simulink model "balance_robot"  (R2024a)
settings: Solver=VariableStepAuto  StartTime=0.0  StopTime=5.2  RelTol=1e-3
values from neighbouring files (symbols this model uses):
  K_cons = zeros(40,6)    [k_calc_chuan.m]    (also in k_calc_chuan_real.m; k_calc_chuanlian_simulink.m)
  X = [x1, x2, x1sq, x2sq, x1x2]    [k_calc_chuan.m]    (also in k_calc_chuan_real.m; k_calc_chuanlian_simulink.m)
undefined symbols (not defined in the file or in its folder): Y, Z
libraries: sm_lib x114, nesl_utility x19, slpidlib x3, simulink x1
(part 3 of 3)

== matlab function balance_robot/RVMC/MATLAB Function ==
  data: phi1 input; L0 output; phi4 input; phi0 output
function [L0,phi0] = L0_PHI0(phi1,phi4)
   % l5=0.108;
   %  l1=0.15;
   %  l2=0.25;
   %  l3=0.25;
   %  l4=0.15;
   %  YD = l4*sin(phi4);
   %  YB = l1*sin(phi1);
   %  XD = l5 + l4*cos(phi4);
   %  XB = l1*cos(phi1); 
   %  lBD = sqrt((XD - XB)*(XD - XB) + (YD - YB)*(YD - YB));
   %  A0 = 2*l2*(XD - XB);
   %  B0 = 2*l2*(YD - YB);
   %  C0 = l2*l2 + lBD*lBD - l3*l3;
   %  phi2 = 2*atan2((B0 + sqrt(A0*A0 + B0*B0 - C0*C0)),(A0 + C0));
   %  XC = l1*cos(phi1) + l2*cos(phi2);
   %  YC = l1*sin(phi1) + l2*sin(phi2);
   %  L0 = sqrt((XC - l5/2)*(XC - l5/2) + YC*YC);
   %  phi0=atan2(YC,(XC-l5/2));
   l1 = 0.075;
   l2 = 0.125;
   l3 = 0.125;
   l4 = 0.075;
   l5 = 0.15;
   XD = l4*cos(phi4);
   YD = l4*sin(phi4);
   XB = l1*cos(phi1);
   YB = l1*sin(phi1);
   lBD = sqrt((XD-XB)^2+(YD-YB)^2);
   A0 = 2*l2*(XD-XB);
   B0 = 2*l2*(YD - YB);
   C0 = l2*l2 + lBD*lBD - l3*l3;
   phi2 = 2*atan2((B0 - sqrt(A0*A0 + B0*B0 - C0*C0)),(A0 + C0));
   XC = (l5/l4)*(l1*cos(phi1) + l2*cos(phi2));
   YC = (l5/l4)*(l1*sin(phi1) + l2*sin(phi2));
   L0 = sqrt(XC*XC + YC*YC);
   phi0=atan2(YC,XC);

   
end

== matlab function balance_robot/Locomotion Controller/MATLAB Function ==
  data: ll input; K output; lr input; K_cons input
function K = I2K(ll, lr, K_cons)
    x = [1, ll, lr, ll^2, lr^2, ll*lr];

    % 初始化反馈矩阵 K（4行10列）
    K = zeros(4, 10);

    % 用 KK 拟合系数矩阵计算每个 K(i,j)
    for i = 1:4
        for j = 1:10
            idx = (i - 1) * 10 + j;      % 找到 K(i,j) 在 KK 中的行号
            coeffs = K_cons(idx, :);         % 拿到该 K(i,j) 的 6 个系数
            K(i, j) = coeffs * x';       % 多项式拟合结果
        end
    end
end

== matlab function balance_robot/RVMC/MATLAB Function1 ==
  data: F0 input; T1 output; Tp input; phi1 input; phi4 input; T2 output
function [T1,T2] = VMC_calc(F0,Tp,phi1,phi4)

   l1 = 0.075;
   l2 = 0.125;
   l3 = 0.125;
   l4 = 0.075;
   l5 = 0.15;

YD = l4*sin(phi4);
YB = l1*sin(phi1);
XD = l4*cos(phi4);
XB = l1*cos(phi1);
lBD = sqrt((XD - XB)*(XD - XB) + (YD - YB)*(YD - YB));
A0 = 2*l2*(XD - XB);
B0 = 2*l2*(YD - YB);
C0 = l2*l2 + lBD*lBD - l3*l3;
phi2 = 2*atan2((B0 - sqrt(A0*A0 + B0*B0 - C0*C0)),A0 + C0);
XC = (l5/l4)*(l1*cos(phi1) + l2*cos(phi2));
YC = (l5/l4)*(l1*sin(phi1) + l2*sin(phi2));
phi3 = atan2(YB-YD+l2*sin(phi2),XB-XD+l2*cos(phi2));
L0 = sqrt(XC*XC + YC*YC);
phi0 = atan2(YC,XC);
j11 = (l1*l5*sin(phi0-phi3)*sin(phi1-phi2))/(l4*sin(phi3-phi2));
j12 = (l1*l5*cos(phi0-phi3)*sin(phi1-phi2))/(L0*l4*sin(phi3-phi2));
j21 = (l5*sin(phi0-phi2)*sin(phi3-phi4))/sin(phi3-phi2);
j22 = (l5*cos(phi0-phi2)*sin(phi3-phi4))/(L0*sin(phi3-phi2));
J = [j11 j12; j21 j22];
F = [F0;Tp];
T = J * F;
T1 = T(1,1);
T2 = T(2,1);

end

== matlab function balance_robot/RVMC/MATLAB Function2 ==
  data: phi1 input; d_phi0 output; phi4 input; d_phi1 input; d_phi4 input
function d_phi0 = D_PHI0(phi1,phi4,d_phi1,d_phi4)
    l1 = 0.075;
   l2 = 0.125;
   l3 = 0.125;
   l4 = 0.075;
   l5 = 0.15;
    d_phi0 =(d_phi1*l5^2*(l2*cos(2*atan2(- (4*l2^2*(l1*cos(phi1) - l4*cos(phi4))^2 + 4*l2^2*(l1*sin(phi1) - l4*sin(phi4))^2 - ((l1*sin(phi1) - l4*sin(phi4))^2 + l2^2 - l3^2 + (l1*cos(phi1) - l4*cos(phi4))^2)^2)^(1/2) - 2*l2*(l1*sin(phi1) - l4*sin(phi4)), (l1*sin(phi1) - l4*sin(phi4))^2 - 2*l2*(l1*cos(phi1) - l4*cos(phi4)) + l2^2 - l3^2 + (l1*cos(phi1) - l4*cos(phi4))^2)) + l1*cos(phi1))^2*((l1*cos(phi1) - (2*l2*cos(2*atan2(- (4*l2^2*(l1*cos(phi1) - l4*cos(phi4))^2 + 4*l2^2*(l1*sin(phi1) - l4*sin(phi4))^2 - ((l1*sin(phi1) - l4*sin(phi4))^2 + l2^2 - l3^2 + (l1*cos(phi1) - l4*cos(phi4))^2)^2)^(1/2) - 2*l2*(l1*sin(phi1) - l4*sin(phi4)), (l1*sin(phi1) - l4*sin(phi4))^2 - 2*l2*(l1*cos(phi1) - l4*cos(phi4)) + l2^2 - l3^2 + (l1*cos(phi1) - l4*cos(phi4))^2))*((real((2*(2*l1*sin(phi1)*(l1*cos(phi1) - l4*cos(phi4)) - 2*l1*cos(phi1)*(l1*sin(phi1) - l4*sin(phi4)))*((l1*sin(phi1) - l4*sin(phi4))^2 + l2^2 - l3^2 + (l1*cos(phi1) - l4*cos(phi4))^2) - 8*l1*l2^2*sin(phi1)*(l1*cos(phi1) - l4*cos(phi4)) + 8*l1*l2^2*cos(phi1)*(l1*sin(phi1) - l4*sin(phi4)))/(4*l2^2*(l1*cos(phi1) - l4*cos(phi4))^2 + 4*l2^2*(l1*sin(phi1) - l4*sin(phi4))^2 - ((l1*sin(phi1) - l4*sin(phi4))^2 + l2^2 - l3^2 + (l1*cos(phi1) - l4*cos(phi4))^2)^2)^(1/2))/2 + 2*l1*l2*cos(phi1))/(imag((4*l2^2*(l1*cos(phi1) - l4*cos(phi4))^2 + 4*l2^2*(l1*sin(phi1) - l4*sin(phi4))^2 - ((l1*sin(phi1) - l4*sin(phi4))^2 + l2^2 - l3^2 + (l1*cos(phi1) - l4*cos(phi4))^2)^2)^(1/2)) + (l1*sin(phi1) - l4*sin(phi4))^2 - 2*l2*(l1*cos(phi1) - l4*cos(phi4)) + l2^2 - l3^2 + (l1*cos(phi1) - l4*cos(phi4))^2) - ((real((4*l2^2*(l1*cos(phi1) - l4*cos(phi4))^2 + 4*l2^2*(l1*sin(phi1) - l4*sin(phi4))^2 - ((l1*sin(phi1) - l4*sin(phi4))^2 + l2^2 - l3^2 + (l1*cos(phi1) - l4*cos(phi4))^2)^2)^(1/2)) + 2*l2*(l1*sin(phi1) - l4*sin(phi4)))*(imag((2*(2*l1*sin(phi1)*(l1*cos(phi1) - l4*cos(phi4)) - 2*l1*cos(phi1)*(l1*sin(phi1) - l4*sin(phi4)))*((l1*sin(phi1) - l4*sin(phi4))^2 + l2^2 - l3^2 + (l1*cos(phi1) - l4*cos(phi4))^2) - 8*l1*l2^2*sin(phi1)*(l1*cos(phi1) - l4*cos(phi4)) + 8*l1*l2^2*cos(phi1)*(l1*sin(phi1) - l4*sin(phi4)))/(4*l2^2*(l1*cos(phi1) - l4*cos(phi4))^2 + 4*l2^2*(l1*sin(phi1) - l4*sin(phi4))^2 - ((l1*sin(phi1) - l4*sin(phi4))^2 + l2^2 - l3^2 + (l1*cos(phi1) - l4*cos(phi4))^2)^2)^(1/2))/2 + 2*l1*l2*sin(phi1) - 2*l1*sin(phi1)*(l1*cos(phi1) - l4*cos(phi4)) + 2*l1*cos(phi1)*(l1*sin(phi1) - l4*sin(phi4))))/(imag((4*l2^2*(l1*cos(phi1) - l4*cos(phi4))^2 + 4*l2^2*(l1*sin(phi1) - l4*sin(phi4))^2 - ((l1*sin(phi1) - l4*sin(phi4))^2 + l2^2 - l3^2 + (l1*cos(phi1) - l4*cos(phi4))^2)^2)^(1/2)) + (l1*sin(phi1) - l4*sin(phi4))^2 - 2*l2*(l1*cos(phi1) - l4*cos(phi4)) + l2^2 - l3^2 + (l1*cos(phi1) - l4*cos(phi4))^2)^2)*(imag((4*l2^2*(l1*cos(phi1) - l4*cos(phi4))^2 + 4*l2^2*(l1*sin(phi1) - l4*sin(phi4))^2 - ((l1*sin(phi1) - l4*sin(phi4))^2 + l2^2 - l3^2 + (l1*cos(phi1) - l4*cos(phi4))^2)^2)^(1/2)) + (l1*sin(phi1) - l4*sin(phi4))^2 - 2*l2*(l1*cos(phi1) - l4*cos(phi4)) + l2^2 - l3^2 + (l1*cos(phi1) - l4*cos(phi4))^2)^2)/((imag((4*l2^2*(l1*cos(phi1) - l4*cos(phi4))^2 + 4*l2^2*(l1*sin(phi1) - l4*sin(phi4))^2 - ((l1*sin(phi1) - l4*sin(phi4))^2 + l2^2 - l3^2 + (l1*cos(phi1) - l4*cos(phi4))^2)^2)^(1/2)) + (l1*sin(phi1) - l4*sin(phi4))^2 - 2*l2*(l1*cos(phi1) - l4*cos(phi4)) + l2^2 - l3^2 + (l1*cos(phi1) - l4*cos(phi4))^2)^2 + (real((4*l2^2*(l1*cos(phi1) - l4*cos(phi4))^2 + 4*l2^2*(l1*sin(phi1) - l4*sin(phi4))^2 - ((l1*sin(phi1) - l4*sin(phi4))^2 + l2^2 - l3^2 + (l1*cos(phi1) - l4*cos(phi4))^2)^2)^(1/2)) + 2*l2*(l1*sin(phi1) - l4*sin(phi4)))^2))/(l2*cos(2*atan2(- (4*l2^2*(l1*cos(phi1) - l4*cos(phi4))^2 + 4*l2^2*(l1*sin(phi1) - l4*sin(phi4))^2 - ((l1*sin(phi1) - l4*sin(phi4))^2 + l2^2 - l3^2 + (l1*cos(phi1) - l4*cos(phi4))^2)^2)^(1/2) - 2*l2*(l1*sin(phi1) - l4*sin(phi4)), (l1*sin(phi1) - l4*sin(phi4))^2 - 2*l2*(l1*cos(phi1) - l4*cos(phi4)) + l2^2 - l3^2 + (l1*cos(phi1) - l4*cos(phi4))^2)) + l1*cos(phi1)) + ((l2*sin(2*atan2(- (4*l2^2*(l1*cos(phi1) - l4*cos(phi4))^2 + 4*l2^2*(l1*sin(phi1) - l4*sin(phi4))^2 - ((l1*sin(phi1) - l4*sin(phi4))^2 + l2^2 - l3^2 + (l1*cos(phi1) - l4*cos(phi4))^2)^2)^(1/2) - 2*l2*(l1*sin(phi1) - l4*sin(phi4)), (l1*sin(phi1) - l4*sin(phi4))^2 - 2*l2*(l1*cos(phi1) - l4*cos(phi4)) + l2^2 - l3^2 + (l1*cos(phi1) - l4*cos(phi4))^2)) + l1*sin(phi1))*(l1*sin(phi1) - (2*l2*sin(2*atan2(- (4*l2^2*(l1*cos(phi1) - l4*cos(phi4))^2 + 4*l2^2*(l1*sin(phi1) - l4*sin(phi4))^2 - ((l1*sin(phi1) - l4*sin(phi4))^2 + l2^2 - l3^2 + (l1*cos(phi1) - l4*cos(phi4))^2)^2)^(1/2) - 2*l2*(l1*sin(phi1) - l4*sin(phi4)), (l1*sin(phi1) - l4*sin(phi4))^2 - 2*l2*(l1*cos(phi1) - l4*cos(phi4)) + l2^2 - l3^2 + (l1*cos(phi1) - l4*cos(phi4))^2))*((real((2*(2*l1*sin(phi1)*(l1*cos(phi1) - l4*cos(phi4)) - 2*l1*cos(phi1)*(l1*sin(phi1) - l4*sin(phi4)))*((l1*sin(phi1) - l4*sin(phi4))^2 + l2^2 - l3^2 + (l1*cos(phi1) - l4*cos(phi4))^2) - 8*l1*l2^2*sin(phi1)*(l1*cos(phi1) - l4*cos(phi4)) + 8*l1*l2^2*cos(phi1)*(l1*sin(phi1) - l4*sin(phi4)))/(4*l2^2*(l1*cos(phi1) - l4*cos(phi4))^2 + 4*l2^2*(l1*sin(phi1) - l4*sin(phi4))^2 - ((l1*sin(phi1) - l4*sin(phi4))^2 + l2^2 - l3^2 + (l1*cos(phi1) - l4*cos(phi4))^2)^2)^(1/2))/2 + 2*l1*l2*cos(phi1))/(imag((4*l2^2*(l1*cos(phi1) - l4*cos(phi4))^2 + 4*l2^2*(l1*sin(phi1) - l4*sin(phi4))^2 - ((l1*sin(phi1) - l4*sin(phi4))^2 + l2^2 - l3^2 + (l1*cos(phi1) - l4*cos(phi4))^2)^2)^(1/2)) + (l1*sin(phi1) - l4*sin(phi4))^2 - 2*l2*(l1*cos(phi1) - l4*cos(phi4)) + l2^2 - l3^2 + (l1*cos(phi1) - l4*cos(phi4))^2) - ((real((4*l2^2*(l1*cos(phi1) - l4*cos(phi4))^2 + 4*l2^2*(l1*sin(phi1) - l4*sin(phi4))^2 - ((l1*sin(phi1) - l4*sin(phi4))^2 + l2^2 - l3^2 + (l1*cos(phi1) - l4*cos(phi4))^2)^2)^(1/2)) + 2*l2*(l1*sin(phi1) - l4*sin(phi4)))*(imag((2*(2*l1*sin(phi1)*(l1*cos(phi1) - l4*cos(phi4)) - 2*l1*cos(phi1)*(l1*sin(phi1) - l4*sin(phi4)))*((l1*sin(phi1) - l4*sin(phi4))^2 + l2^2 - l3^2 + (l1*cos(phi1) - l4*cos(phi4))^2) - 8*l1*l2^2*sin(phi1)*(l1*cos(phi1) - l4*cos(phi4)) + 8*l1*l2^2*cos(phi1)*(l1*sin(phi1) - l4*sin(phi4)))/(4*l2^2*(l1*cos(phi1) - l4*cos(phi4))^2 + 4*l2^2*(l1*sin(phi1) - l4*sin(phi4))^2 - ((l1*sin(phi1) - l4*sin(phi4))^2 + l2^2 - l3^2 + (l1*cos(phi1) - l4*cos(phi4))^2)^2)^(1/2))/2 + 2*l1*l2*sin(phi1) - 2*l1*sin(phi1)*(l1*cos(phi1) - l4*cos(phi4)) + 2*l1*cos(phi1)*(l1*sin(phi1) - l4*sin(phi4))))/(imag((4*l2^2*(l1*cos(phi1) - l4*cos(phi4))^2 + 4*l2^2*(l1*sin(phi1) - l4*sin(phi4))^2 - ((l1*sin(phi1) - l4*sin(phi4))^2 + l2^2 - l3^2 + (l1*cos(phi1) - l4*cos(phi4))^2)^2)^(1/2)) + (l1*sin(phi1) - l4*sin(phi4))^2 - 2*l2*(l1*cos(phi1) - l4*cos(phi4)) + l2^2 - l3^2 + (l1*cos(phi1) - l4*cos(phi4))^2)^2)*(imag((4*l2^2*(l1*cos(phi1) - l4*cos(phi4))^2 + 4*l2^2*(l1*sin(phi1) - l4*sin(phi4))^2 - ((l1*sin(phi1) - l4*sin(phi4))^2 + l2^2 - l3^2 + (l1*cos(phi1) - l4*cos(phi4))^2)^2)^(1/2)) + (l1*sin(phi1) - l4*sin(phi4))^2 - 2*l2*(l1*cos(phi1) - l4*cos(phi4)) + l2^2 - l3^2 + (l1*cos(phi1) - l4*cos(phi4))^2)^2)/((imag((4*l2^2*(l1*cos(phi1) - l4*cos(phi4))^2 + 4*l2^2*(l1*sin(phi1) - l4*sin(phi4))^2 - ((l1*sin(phi1) - l4*sin(phi4))^2 + l2^2 - l3^2 + (l1*cos(phi1) - l4*cos(phi4))^2)^2)^(1/2)) + (l1*sin(phi1) - l4*sin(phi4))^2 - 2*l2*(l1*cos(phi1) - l4*cos(phi4)) + l2^2 - l3^2 + (l1*cos(phi1) - l4*cos(phi4))^2)^2 + (real((4*l2^2*(l1*cos(phi1) - l4*cos(phi4))^2 + 4*l2^2*(l1*sin(phi1) - l4*sin(phi4))^2 - ((l1*sin(phi1) - l4*sin(phi4))^2 + l2^2 - l3^2 + (l1*cos(phi1) - l4*cos(phi4))^2)^2)^(1/2)) + 2*l2*(l1*sin(phi1) - l4*sin(phi4)))^2)))/(l2*cos(2*atan2(- (4*l2^2*(l1*cos(phi1) - l4*cos(phi4))^2 + 4*l2^2*(l1*sin(phi1) - l4*sin(phi4))^2 - ((l1*sin(phi1) - l4*sin(phi4))^2 + l2^2 - l3^2 + (l1*cos(phi1) - l4*cos(phi4))^2)^2)^(1/2) - 2*l2*(l1*sin(phi1) - l4*sin(phi4)), (l1*sin(phi1) - l4*sin(phi4))^2 - 2*l2*(l1*cos(phi1) - l4*cos(phi4)) + l2^2 - l3^2 + (l1*cos(phi1) - l4*cos(phi4))^2)) + l1*cos(phi1))^2))/(l4^2*((l5^2*(l2*cos(2*atan2(- (4*l2^2*(l1*cos(phi1) - l4*cos(phi4))^2 + 4*l2^2*(l1*sin(phi1) - l4*sin(phi4))^2 - ((l1*sin(phi1) - l4*sin(phi4))^2 + l2^2 - l3^2 + (l1*cos(phi1) - l4*cos(phi4))^2)^2)^(1/2) - 2*l2*(l1*sin(phi1) - l4*sin(phi4)), (l1*sin(phi1) - l4*sin(phi4))^2 - 2*l2*(l1*cos(phi1) - l4*cos(phi4)) + l2^2 - l3^2 + (l1*cos(phi1) - l4*cos(phi4))^2)) + l1*cos(phi1))^2)/l4^2 + (l5^2*(l2*sin(2*atan2(- (4*l2^2*(l1*cos(phi1) - l4*cos(phi4))^2 + 4*l2^2*(l1*sin(phi1) - l4*sin(phi4))^2 - ((l1*sin(phi1) - l4*sin(phi4))^2 + l2^2 - l3^2 + (l1*cos(phi1) - l4*cos(phi4))^2)^2)^(1/2) - 2*l2*(l1*sin(phi1) - l4*sin(phi4)), (l1*sin(phi1) - l4*sin(phi4))^2 - 2*l2*(l1*cos(phi1) - l4*cos(phi4)) + l2^2 - l3^2 + (l1*cos(phi1) - l4*cos(phi4))^2)) + l1*sin(phi1))^2)/l4^2)) + (d_phi4*l5^2*(l2*cos(2*atan2(- (4*l2^2*(l1*cos(phi1) - l4*cos(phi4))^2 + 4*l2^2*(l1*sin(phi1) - l4*sin(phi4))^2 - ((l1*sin(phi1) - l4*sin(phi4))^2 + l2^2 - l3^2 + (l1*cos(phi1) - l4*cos(phi4))^2)^2)^(1/2) - 2*l2*(l1*sin(phi1) - l4*sin(phi4)), (l1*sin(phi1) - l4*sin(phi4))^2 - 2*l2*(l1*cos(phi1) - l4*cos(phi4)) + l2^2 - l3^2 + (l1*cos(phi1) - l4*cos(phi4))^2)) + l1*cos(phi1))^2*((2*l2*cos(2*atan2(- (4*l2^2*(l1*cos(phi1) - l4*cos(phi4))^2 + 4*l2^2*(l1*sin(phi1) - l4*sin(phi4))^2 - ((l1*sin(phi1) - l4*sin(phi4))^2 + l2^2 - l3^2 + (l1*cos(phi1) - l4*cos(phi4))^2)^2)^(1/2) - 2*l2*(l1*sin(phi1) - l4*sin(phi4)), (l1*sin(phi1) - l4*sin(phi4))^2 - 2*l2*(l1*cos(phi1) - l4*cos(phi4)) + l2^2 - l3^2 + (l1*cos(phi1) - l4*cos(phi4))^2))*((real((2*(2*l4*sin(phi4)*(l1*cos(phi1) - l4*cos(phi4)) - 2*l4*cos(phi4)*(l1*sin(phi1) - l4*sin(phi4)))*((l1*sin(phi1) - l4*sin(phi4))^2 + l2^2 - l3^2 + (l1*cos(phi1) - l4*cos(phi4))^2) - 8*l2^2*l4*sin(phi4)*(l1*cos(phi1) - l4*cos(phi4)) + 8*l2^2*l4*cos(phi4)*(l1*sin(phi1) - l4*sin(phi4)))/(4*l2^2*(l1*cos(phi1) - l4*cos(phi4))^2 + 4*l2^2*(l1*sin(phi1) - l4*sin(phi4))^2 - ((l1*sin(phi1) - l4*sin(phi4))^2 + l2^2 - l3^2 + (l1*cos(phi1) - l4*cos(phi4))^2)^2)^(1/2))/2 + 2*l2*l4*cos(phi4))/(imag((4*l2^2*(l1*cos(phi1) - l4*cos(phi4))^2 + 4*l2^2*(l1*sin(phi1) - l4*sin(phi4))^2 - ((l1*sin(phi1) - l4*sin(phi4))^2 + l2^2 - l3^2 + (l1*cos(phi1) - l4*cos(phi4))^2)^2)^(1/2)) + (l1*sin(phi1) - l4*sin(phi4))^2 - 2*l2*(l1*cos(phi1) - l4*cos(phi4)) + l2^2 - l3^2 + (l1*cos(phi1) - l4*cos(phi4))^2) - ((real((4*l2^2*(l1*cos(phi1) - l4*cos(phi4))^2 + 4*l2^2*(l1*sin(phi1) - l4*sin(phi4))^2 - ((l1*sin(phi1) - l4*sin(phi4))^2 + l2^2 - l3^2 + (l1*cos(phi1) - l4*cos(phi4))^2)^2)^(1/2)) + 2*l2*(l1*sin(phi1) - l4*sin(phi4)))*(imag((2*(2*l4*sin(phi4)*(l1*cos(phi1) - l4*cos(phi4)) - 2*l4*cos(phi4)*(l1*sin(phi1) - l4*sin(phi4)))*((l1*sin(phi1) - l4*sin(phi4))^2 + l2^2 - l3^2 + (l1*cos(phi1) - l4*cos(phi4))^2) - 8*l2^2*l4*sin(phi4)*(l1*cos(phi1) - l4*cos(phi4)) + 8*l2^2*l4*cos(phi4)*(l1*sin(phi1) - l4*sin(phi4)))/(4*l2^2*(l1*cos(phi1) - l4*cos(phi4))^2 + 4*l2^2*(l1*sin(phi1) - l4*sin(phi4))^2 - ((l1*sin(phi1) - l4*sin(phi4))^2 + l2^2 - l3^2 + (l1*cos(phi1) - l4*cos(phi4))^2)^2)^(1/2))/2 + 2*l2*l4*sin(phi4) - 2*l4*sin(phi4)*(l1*cos(phi1) - l4*cos(phi4)) + 2*l4*cos(phi4)*(l1*sin(phi1) - l4*sin(phi4))))/(imag((4*l2^2*(l1*cos(phi1) - l4*cos(phi4))^2 + 4*l2^2*(l1*sin(phi1) - l4*sin(phi4))^2 - ((l1*sin(phi1) - l4*sin(phi4))^2 + l2^2 - l3^2 + (l1*cos(phi1) - l4*cos(phi4))^2)^2)^(1/2)) + (l1*sin(phi1) - l4*sin(phi4))^2 - 2*l2*(l1*cos(phi1) - l4*cos(phi4)) + l2^2 - l3^2 + (l1*cos(phi1) - l4*cos(phi4))^2)^2)*(imag((4*l2^2*(l1*cos(phi1) - l4*cos(phi4))^2 + 4*l2^2*(l1*sin(phi1) - l4*sin(phi4))^2 - ((l1*sin(phi1) - l4*sin(phi4))^2 + l2^2 - l3^2 + (l1*cos(phi1) - l4*cos(phi4))^2)^2)^(1/2)) + (l1*sin(phi1) - l4*sin(phi4))^2 - 2*l2*(l1*cos(phi1) - l4*cos(phi4)) + l2^2 - l3^2 + (l1*cos(phi1) - l4*cos(phi4))^2)^2)/((l2*cos(2*atan2(- (4*l2^2*(l1*cos(phi1) - l4*cos(phi4))^2 + 4*l2^2*(l1*sin(phi1) - l4*sin(phi4))^2 - ((l1*sin(phi1) - l4*sin(phi4))^2 + l2^2 - l3^2 + (l1*cos(phi1) - l4*cos(phi4))^2)^2)^(1/2) - 2*l2*(l1*sin(phi1) - l4*sin(phi4)), (l1*sin(phi1) - l4*sin(phi4))^2 - 2*l2*(l1*cos(phi1) - l4*cos(phi4)) + l2^2 - l3^2 + (l1*cos(phi1) - l4*cos(phi4))^2)) + l1*cos(phi1))*((imag((4*l2^2*(l1*cos(phi1) - l4*cos(phi4))^2 + 4*l2^2*(l1*sin(phi1) - l4*sin(phi4))^2 - ((l1*sin(phi1) - l4*sin(phi4))^2 + l2^2 - l3^2 + (l1*cos(phi1) - l4*cos(phi4))^2)^2)^(1/2)) + (l1*sin(phi1) - l4*sin(phi4))^2 - 2*l2*(l1*cos(phi1) - l4*cos(phi4)) + l2^2 - l3^2 + (l1*cos(phi1) - l4*cos(phi4))^2)^2 + (real((4*l2^2*(l1*cos(phi1) - l4*cos(phi4))^2 + 4*l2^2*(l1*sin(phi1) - l4*sin(phi4))^2 - ((l1*sin(phi1) - l4*sin(phi4))^2 + l2^2 - l3^2 + (l1*cos(phi1) - l4*cos(phi4))^2)^2)^(1/2)) + 2*l2*(l1*sin(phi1) - l4*sin(phi4)))^2)) + (2*l2*sin(2*atan2(- (4*l2^2*(l1*cos(phi1) - l4*cos(phi4))^2 + 4*l2^2*(l1*sin(phi1) - l4*sin(phi4))^2 - ((l1*sin(phi1) - l4*sin(phi4))^2 + l2^2 - l3^2 + (l1*cos(phi1) - l4*cos(phi4))^2)^2)^(1/2) - 2*l2*(l1*sin(phi1) - l4*sin(phi4)), (l1*sin(phi1) - l4*sin(phi4))^2 - 2*l2*(l1*cos(phi1) - l4*cos(phi4)) + l2^2 - l3^2 + (l1*cos(phi1) - l4*cos(phi4))^2))*(l2*sin(2*atan2(- (4*l2^2*(l1*cos(phi1) - l4*cos(phi4))^2 + 4*l2^2*(l1*sin(phi1) - l4*sin(phi4))^2 - ((l1*sin(phi1) - l4*sin(phi4))^2 + l2^2 - l3^2 + (l1*cos(phi1) - l4*cos(phi4))^2)^2)^(1/2) - 2*l2*(l1*sin(phi1) - l4*sin(phi4)), (l1*sin(phi1) - l4*sin(phi4))^2 - 2*l2*(l1*cos(phi1) - l4*cos(phi4)) + l2^2 - l3^2 + (l1*cos(phi1) - l4*cos(phi4))^2)) + l1*sin(phi1))*((real((2*(2*l4*sin(phi4)*(l1*cos(phi1) - l4*cos(phi4)) - 2*l4*cos(phi4)*(l1*sin(phi1) - l4*sin(phi4)))*((l1*sin(phi1) - l4*sin(phi4))^2 + l2^2 - l3^2 + (l1*cos(phi1) - l4*cos(phi4))^2) - 8*l2^2*l4*sin(phi4)*(l1*cos(phi1) - l4*cos(phi4)) + 8*l2^2*l4*cos(phi4)*(l1*sin(phi1) - l4*sin(phi4)))/(4*l2^2*(l1*cos(phi1) - l4*cos(phi4))^2 + 4*l2^2*(l1*sin(phi1) - l4*sin(phi4))^2 - ((l1*sin(phi1) - l4*sin(phi4))^2 + l2^2 - l3^2 + (l1*cos(phi1) - l4*cos(phi4))^2)^2)^(1/2))/2 + 2*l2*l4*cos(phi4))/(imag((4*l2^2*(l1*cos(phi1) - l4*cos(phi4))^2 + 4*l2^2*(l1*sin(phi1) - l4*sin(phi4))^2 - ((l1*sin(phi1) - l4*sin(phi4))^2 + l2^2 - l3^2 + (l1*cos(phi1) - l4*cos(phi4))^2)^2)^(1/2)) + (l1*sin(phi1) - l4*sin(phi4))^2 - 2*l2*(l1*cos(phi1) - l4*cos(phi4)) + l2^2 - l3^2 + (l1*cos(phi1) - l4*cos(phi4))^2) - ((real((4*l2^2*(l1*cos(phi1) - l4*cos(phi4))^2 + 4*l2^2*(l1*sin(phi1) - l4*sin(phi4))^2 - ((l1*sin(phi1) - l4*sin(phi4))^2 + l2^2 - l3^2 + (l1*cos(phi1) - l4*cos(phi4))^2)^2)^(1/2)) + 2*l2*(l1*sin(phi1) - l4*sin(phi4)))*(imag((2*(2*l4*sin(phi4)*(l1*cos(phi1) - l4*cos(phi4)) - 2*l4*cos(phi4)*(l1*sin(phi1) - l4*sin(phi4)))*((l1*sin(phi1) - l4*sin(phi4))^2 + l2^2 - l3^2 + (l1*cos(phi1) - l4*cos(phi4))^2) - 8*l2^2*l4*sin(phi4)*(l1*cos(phi1) - l4*cos(phi4)) + 8*l2^2*l4*cos(phi4)*(l1*sin(phi1) - l4*sin(phi4)))/(4*l2^2*(l1*cos(phi1) - l4*cos(phi4))^2 + 4*l2^2*(l1*sin(phi1) - l4*sin(phi4))^2 - ((l1*sin(phi1) - l4*sin(phi4))^2 + l2^2 - l3^2 + (l1*cos(phi1) - l4*cos(phi4))^2)^2)^(1/2))/2 + 2*l2*l4*sin(phi4) - 2*l4*sin(phi4)*(l1*cos(phi1) - l4*cos(phi4)) + 2*l4*cos(phi4)*(l1*sin(phi1) - l4*sin(phi4))))/(imag((4*l2^2*(l1*cos(phi1) - l4*cos(phi4))^2 + 4*l2^2*(l1*sin(phi1) - l4*sin(phi4))^2 - ((l1*sin(phi1) - l4*sin(phi4))^2 + l2^2 - l3^2 + (l1*cos(phi1) - l4*cos(phi4))^2)^2)^(1/2)) + (l1*sin(phi1) - l4*sin(phi4))^2 - 2*l2*(l1*cos(phi1) - l4*cos(phi4)) + l2^2 - l3^2 + (l1*cos(phi1) - l4*cos(phi4))^2)^2)*(imag((4*l2^2*(l1*cos(phi1) - l4*cos(phi4))^2 + 4*l2^2*(l1*sin(phi1) - l4*sin(phi4))^2 - ((l1*sin(phi1) - l4*sin(phi4))^2 + l2^2 - l3^2 + (l1*cos(phi1) - l4*cos(phi4))^2)^2)^(1/2)) + (l1*sin(phi1) - l4*sin(phi4))^2 - 2*l2*(l1*cos(phi1) - l4*cos(phi4)) + l2^2 - l3^2 + (l1*cos(phi1) - l4*cos(phi4))^2)^2)/((l2*cos(2*atan2(- (4*l2^2*(l1*cos(phi1) - l4*cos(phi4))^2 + 4*l2^2*(l1*sin(phi1) - l4*sin(phi4))^2 - ((l1*sin(phi1) - l4*sin(phi4))^2 + l2^2 - l3^2 + (l1*cos(phi1) - l4*cos(phi4))^2)^2)^(1/2) - 2*l2*(l1*sin(phi1) - l4*sin(phi4)), (l1*sin(phi1) - l4*sin(phi4))^2 - 2*l2*(l1*cos(phi1) - l4*cos(phi4)) + l2^2 - l3^2 + (l1*cos(phi1) - l4*cos(phi4))^2)) + l1*cos(phi1))^2*((imag((4*l2^2*(l1*cos(phi1) - l4*cos(phi4))^2 + 4*l2^2*(l1*sin(phi1) - l4*sin(phi4))^2 - ((l1*sin(phi1) - l4*sin(phi4))^2 + l2^2 - l3^2 + (l1*cos(phi1) - l4*cos(phi4))^2)^2)^(1/2)) + (l1*sin(phi1) - l4*sin(phi4))^2 - 2*l2*(l1*cos(phi1) - l4*cos(phi4)) + l2^2 - l3^2 + (l1*cos(phi1) - l4*cos(phi4))^2)^2 + (real((4*l2^2*(l1*cos(phi1) - l4*cos(phi4))^2 + 4*l2^2*(l1*sin(phi1) - l4*sin(phi4))^2 - ((l1*sin(phi1) - l4*sin(phi4))^2 + l2^2 - l3^2 + (l1*cos(phi1) - l4*cos(phi4))^2)^2)^(1/2)) + 2*l2*(l1*sin(phi1) - l4*sin(phi4)))^2))))/(l4^2*((l5^2*(l2*cos(2*atan2(- (4*l2^2*(l1*cos(phi1) - l4*cos(phi4))^2 + 4*l2^2*(l1*sin(phi1) - l4*sin(phi4))^2 - ((l1*sin(phi1) - l4*sin(phi4))^2 + l2^2 - l3^2 + (l1*cos(phi1) - l4*cos(phi4))^2)^2)^(1/2) - 2*l2*(l1*sin(phi1) - l4*sin(phi4)), (l1*sin(phi1) - l4*sin(phi4))^2 - 2*l2*(l1*cos(phi1) - l4*cos(phi4)) + l2^2 - l3^2 + (l1*cos(phi1) - l4*cos(phi4))^2)) + l1*cos(phi1))^2)/l4^2 + (l5^2*(l2*sin(2*atan2(- (4*l2^2*(l1*cos(phi1) - l4*cos(phi4))^2 + 4*l2^2*(l1*sin(phi1) - l4*sin(phi4))^2 - ((l1*sin(phi1) - l4*sin(phi4))^2 + l2^2 - l3^2 + (l1*cos(phi1) - l4*cos(phi4))^2)^2)^(1/2) - 2*l2*(l1*sin(phi1) - l4*sin(phi4)), (l1*sin(phi1) - l4*sin(phi4))^2 - 2*l2*(l1*cos(phi1) - l4*cos(phi4)) + l2^2 - l3^2 + (l1*cos(phi1) - l4*cos(phi4))^2)) + l1*sin(phi1))^2)/l4^2));
 
end

== matlab function balance_robot/LVMC/MATLAB Function ==
  data: phi1 input; L0 output; phi4 input; phi0 output
function [L0,phi0] = L0_PHI0(phi1,phi4)
   % l5=0.108;
   %  l1=0.15;
   %  l2=0.25;
   %  l3=0.25;
   %  l4=0.15;
   %  YD = l4*sin(phi4);
   %  YB = l1*sin(phi1);
   %  XD = l5 + l4*cos(phi4);
   %  XB = l1*cos(phi1); 
   %  lBD = sqrt((XD - XB)*(XD - XB) + (YD - YB)*(YD - YB));
   %  A0 = 2*l2*(XD - XB);
   %  B0 = 2*l2*(YD - YB);
   %  C0 = l2*l2 + lBD*lBD - l3*l3;
   %  phi2 = 2*atan2((B0 + sqrt(A0*A0 + B0*B0 - C0*C0)),(A0 + C0));
   %  XC = l1*cos(phi1) + l2*cos(phi2);
   %  YC = l1*sin(phi1) + l2*sin(phi2);
   %  L0 = sqrt((XC - l5/2)*(XC - l5/2) + YC*YC);
   %  phi0=atan2(YC,(XC-l5/2));
   l1 = 0.075;
   l2 = 0.125;
   l3 = 0.125;
   l4 = 0.075;
   l5 = 0.15;
   XD = l4*cos(phi4);
   YD = l4*sin(phi4);
   XB = l1*cos(phi1);
   YB = l1*sin(phi1);
   lBD = sqrt((XD-XB)^2+(YD-YB)^2);
   A0 = 2*l2*(XD-XB);
   B0 = 2*l2*(YD - YB);
   C0 = l2*l2 + lBD*lBD - l3*l3;
   phi2 = 2*atan2((B0 - sqrt(A0*A0 + B0*B0 - C0*C0)),(A0 + C0));
   XC = l5/l4*(l1*cos(phi1) + l2*cos(phi2));
   YC = l5/l4*(l1*sin(phi1) + l2*sin(phi2));
   L0 = sqrt(XC*XC + YC*YC);
   phi0=atan2(YC,XC);

   
end

== matlab function balance_robot/LVMC/MATLAB Function1 ==
  data: F0 input; T1 output; Tp input; phi1 input; phi4 input; T2 output
function [T1,T2] = VMC_calc(F0,Tp,phi1,phi4)

   l1 = 0.075;
   l2 = 0.125;
   l3 = 0.125;
   l4 = 0.075;
   l5 = 0.15;

YD = l4*sin(phi4);
YB = l1*sin(phi1);
XD = l4*cos(phi4);
XB = l1*cos(phi1);
lBD = sqrt((XD - XB)*(XD - XB) + (YD - YB)*(YD - YB));
A0 = 2*l2*(XD - XB);
B0 = 2*l2*(YD - YB);
C0 = l2*l2 + lBD*lBD - l3*l3;
phi2 = 2*atan2((B0 - sqrt(A0*A0 + B0*B0 - C0*C0)),A0 + C0);
XC = l5/l4*(l1*cos(phi1) + l2*cos(phi2));
YC = l5/l4*(l1*sin(phi1) + l2*sin(phi2));
phi3 = atan2(YB-YD+l2*sin(phi2),XB-XD+l2*cos(phi2));
L0 = sqrt(XC*XC + YC*YC);
phi0 = atan2(YC,XC);
j11 = (l1*l5*sin(phi0-phi3)*sin(phi1-phi2))/(l4*sin(phi3-phi2));
j12 = (l1*l5*cos(phi0-phi3)*sin(phi1-phi2))/(L0*l4*sin(phi3-phi2));
j21 = (l5*sin(phi0-phi2)*sin(phi3-phi4))/sin(phi3-phi2);
j22 = (l5*cos(phi0-phi2)*sin(phi3-phi4))/(L0*sin(phi3-phi2));
J = [j11 j12; j21 j22];
F = [F0;Tp];
T = J * F;
T1 = T(1,1);
T2 = T(2,1);

end

== matlab function balance_robot/LVMC/MATLAB Function2 ==
  data: phi1 input; d_phi0 output; phi4 input; d_phi1 input; d_phi4 input
function d_phi0 = D_PHI0(phi1,phi4,d_phi1,d_phi4)
    l1 = 0.075;
   l2 = 0.125;
   l3 = 0.125;
   l4 = 0.075;
   l5 = 0.15;
    d_phi0 =(d_phi1*l5^2*(l2*cos(2*atan2(- (4*l2^2*(l1*cos(phi1) - l4*cos(phi4))^2 + 4*l2^2*(l1*sin(phi1) - l4*sin(phi4))^2 - ((l1*sin(phi1) - l4*sin(phi4))^2 + l2^2 - l3^2 + (l1*cos(phi1) - l4*cos(phi4))^2)^2)^(1/2) - 2*l2*(l1*sin(phi1) - l4*sin(phi4)), (l1*sin(phi1) - l4*sin(phi4))^2 - 2*l2*(l1*cos(phi1) - l4*cos(phi4)) + l2^2 - l3^2 + (l1*cos(phi1) - l4*cos(phi4))^2)) + l1*cos(phi1))^2*((l1*cos(phi1) - (2*l2*cos(2*atan2(- (4*l2^2*(l1*cos(phi1) - l4*cos(phi4))^2 + 4*l2^2*(l1*sin(phi1) - l4*sin(phi4))^2 - ((l1*sin(phi1) - l4*sin(phi4))^2 + l2^2 - l3^2 + (l1*cos(phi1) - l4*cos(phi4))^2)^2)^(1/2) - 2*l2*(l1*sin(phi1) - l4*sin(phi4)), (l1*sin(phi1) - l4*sin(phi4))^2 - 2*l2*(l1*cos(phi1) - l4*cos(phi4)) + l2^2 - l3^2 + (l1*cos(phi1) - l4*cos(phi4))^2))*((real((2*(2*l1*sin(phi1)*(l1*cos(phi1) - l4*cos(phi4)) - 2*l1*cos(phi1)*(l1*sin(phi1) - l4*sin(phi4)))*((l1*sin(phi1) - l4*sin(phi4))^2 + l2^2 - l3^2 + (l1*cos(phi1) - l4*cos(phi4))^2) - 8*l1*l2^2*sin(phi1)*(l1*cos(phi1) - l4*cos(phi4)) + 8*l1*l2^2*cos(phi1)*(l1*sin(phi1) - l4*sin(phi4)))/(4*l2^2*(l1*cos(phi1) - l4*cos(phi4))^2 + 4*l2^2*(l1*sin(phi1) - l4*sin(phi4))^2 - ((l1*sin(phi1) - l4*sin(phi4))^2 + l2^2 - l3^2 + (l1*cos(phi1) - l4*cos(phi4))^2)^2)^(1/2))/2 + 2*l1*l2*cos(phi1))/(imag((4*l2^2*(l1*cos(phi1) - l4*cos(phi4))^2 + 4*l2^2*(l1*sin(phi1) - l4*sin(phi4))^2 - ((l1*sin(phi1) - l4*sin(phi4))^2 + l2^2 - l3^2 + (l1*cos(phi1) - l4*cos(phi4))^2)^2)^(1/2)) + (l1*sin(phi1) - l4*sin(phi4))^2 - 2*l2*(l1*cos(phi1) - l4*cos(phi4)) + l2^2 - l3^2 + (l1*cos(phi1) - l4*cos(phi4))^2) - ((real((4*l2^2*(l1*cos(phi1) - l4*cos(phi4))^2 + 4*l2^2*(l1*sin(phi1) - l4*sin(phi4))^2 - ((l1*sin(phi1) - l4*sin(phi4))^2 + l2^2 - l3^2 + (l1*cos(phi1) - l4*cos(phi4))^2)^2)^(1/2)) + 2*l2*(l1*sin(phi1) - l4*sin(phi4)))*(imag((2*(2*l1*sin(phi1)*(l1*cos(phi1) - l4*cos(phi4)) - 2*l1*cos(phi1)*(l1*sin(phi1) - l4*sin(phi4)))*((l1*sin(phi1) - l4*sin(phi4))^2 + l2^2 - l3^2 + (l1*cos(phi1) - l4*cos(phi4))^2) - 8*l1*l2^2*sin(phi1)*(l1*cos(phi1) - l4*cos(phi4)) + 8*l1*l2^2*cos(phi1)*(l1*sin(phi1) - l4*sin(phi4)))/(4*l2^2*(l1*cos(phi1) - l4*cos(phi4))^2 + 4*l2^2*(l1*sin(phi1) - l4*sin(phi4))^2 - ((l1*sin(phi1) - l4*sin(phi4))^2 + l2^2 - l3^2 + (l1*cos(phi1) - l4*cos(phi4))^2)^2)^(1/2))/2 + 2*l1*l2*sin(phi1) - 2*l1*sin(phi1)*(l1*cos(phi1) - l4*cos(phi4)) + 2*l1*cos(phi1)*(l1*sin(phi1) - l4*sin(phi4))))/(imag((4*l2^2*(l1*cos(phi1) - l4*cos(phi4))^2 + 4*l2^2*(l1*sin(phi1) - l4*sin(phi4))^2 - ((l1*sin(phi1) - l4*sin(phi4))^2 + l2^2 - l3^2 + (l1*cos(phi1) - l4*cos(phi4))^2)^2)^(1/2)) + (l1*sin(phi1) - l4*sin(phi4))^2 - 2*l2*(l1*cos(phi1) - l4*cos(phi4)) + l2^2 - l3^2 + (l1*cos(phi1) - l4*cos(phi4))^2)^2)*(imag((4*l2^2*(l1*cos(phi1) - l4*cos(phi4))^2 + 4*l2^2*(l1*sin(phi1) - l4*sin(phi4))^2 - ((l1*sin(phi1) - l4*sin(phi4))^2 + l2^2 - l3^2 + (l1*cos(phi1) - l4*cos(phi4))^2)^2)^(1/2)) + (l1*sin(phi1) - l4*sin(phi4))^2 - 2*l2*(l1*cos(phi1) - l4*cos(phi4)) + l2^2 - l3^2 + (l1*cos(phi1) - l4*cos(phi4))^2)^2)/((imag((4*l2^2*(l1*cos(phi1) - l4*cos(phi4))^2 + 4*l2^2*(l1*sin(phi1) - l4*sin(phi4))^2 - ((l1*sin(phi1) - l4*sin(phi4))^2 + l2^2 - l3^2 + (l1*cos(phi1) - l4*cos(phi4))^2)^2)^(1/2)) + (l1*sin(phi1) - l4*sin(phi4))^2 - 2*l2*(l1*cos(phi1) - l4*cos(phi4)) + l2^2 - l3^2 + (l1*cos(phi1) - l4*cos(phi4))^2)^2 + (real((4*l2^2*(l1*cos(phi1) - l4*cos(phi4))^2 + 4*l2^2*(l1*sin(phi1) - l4*sin(phi4))^2 - ((l1*sin(phi1) - l4*sin(phi4))^2 + l2^2 - l3^2 + (l1*cos(phi1) - l4*cos(phi4))^2)^2)^(1/2)) + 2*l2*(l1*sin(phi1) - l4*sin(phi4)))^2))/(l2*cos(2*atan2(- (4*l2^2*(l1*cos(phi1) - l4*cos(phi4))^2 + 4*l2^2*(l1*sin(phi1) - l4*sin(phi4))^2 - ((l1*sin(phi1) - l4*sin(phi4))^2 + l2^2 - l3^2 + (l1*cos(phi1) - l4*cos(phi4))^2)^2)^(1/2) - 2*l2*(l1*sin(phi1) - l4*sin(phi4)), (l1*sin(phi1) - l4*sin(phi4))^2 - 2*l2*(l1*cos(phi1) - l4*cos(phi4)) + l2^2 - l3^2 + (l1*cos(phi1) - l4*cos(phi4))^2)) + l1*cos(phi1)) + ((l2*sin(2*atan2(- (4*l2^2*(l1*cos(phi1) - l4*cos(phi4))^2 + 4*l2^2*(l1*sin(phi1) - l4*sin(phi4))^2 - ((l1*sin(phi1) - l4*sin(phi4))^2 + l2^2 - l3^2 + (l1*cos(phi1) - l4*cos(phi4))^2)^2)^(1/2) - 2*l2*(l1*sin(phi1) - l4*sin(phi4)), (l1*sin(phi1) - l4*sin(phi4))^2 - 2*l2*(l1*cos(phi1) - l4*cos(phi4)) + l2^2 - l3^2 + (l1*cos(phi1) - l4*cos(phi4))^2)) + l1*sin(phi1))*(l1*sin(phi1) - (2*l2*sin(2*atan2(- (4*l2^2*(l1*cos(phi1) - l4*cos(phi4))^2 + 4*l2^2*(l1*sin(phi1) - l4*sin(phi4))^2 - ((l1*sin(phi1) - l4*sin(phi4))^2 + l2^2 - l3^2 + (l1*cos(phi1) - l4*cos(phi4))^2)^2)^(1/2) - 2*l2*(l1*sin(phi1) - l4*sin(phi4)), (l1*sin(phi1) - l4*sin(phi4))^2 - 2*l2*(l1*cos(phi1) - l4*cos(phi4)) + l2^2 - l3^2 + (l1*cos(phi1) - l4*cos(phi4))^2))*((real((2*(2*l1*sin(phi1)*(l1*cos(phi1) - l4*cos(phi4)) - 2*l1*cos(phi1)*(l1*sin(phi1) - l4*sin(phi4)))*((l1*sin(phi1) - l4*sin(phi4))^2 + l2^2 - l3^2 + (l1*cos(phi1) - l4*cos(phi4))^2) - 8*l1*l2^2*sin(phi1)*(l1*cos(phi1) - l4*cos(phi4)) + 8*l1*l2^2*cos(phi1)*(l1*sin(phi1) - l4*sin(phi4)))/(4*l2^2*(l1*cos(phi1) - l4*cos(phi4))^2 + 4*l2^2*(l1*sin(phi1) - l4*sin(phi4))^2 - ((l1*sin(phi1) - l4*sin(phi4))^2 + l2^2 - l3^2 + (l1*cos(phi1) - l4*cos(phi4))^2)^2)^(1/2))/2 + 2*l1*l2*cos(phi1))/(imag((4*l2^2*(l1*cos(phi1) - l4*cos(phi4))^2 + 4*l2^2*(l1*sin(phi1) - l4*sin(phi4))^2 - ((l1*sin(phi1) - l4*sin(phi4))^2 + l2^2 - l3^2 + (l1*cos(phi1) - l4*cos(phi4))^2)^2)^(1/2)) + (l1*sin(phi1) - l4*sin(phi4))^2 - 2*l2*(l1*cos(phi1) - l4*cos(phi4)) + l2^2 - l3^2 + (l1*cos(phi1) - l4*cos(phi4))^2) - ((real((4*l2^2*(l1*cos(phi1) - l4*cos(phi4))^2 + 4*l2^2*(l1*sin(phi1) - l4*sin(phi4))^2 - ((l1*sin(phi1) - l4*sin(phi4))^2 + l2^2 - l3^2 + (l1*cos(phi1) - l4*cos(phi4))^2)^2)^(1/2)) + 2*l2*(l1*sin(phi1) - l4*sin(phi4)))*(imag((2*(2*l1*sin(phi1)*(l1*cos(phi1) - l4*cos(phi4)) - 2*l1*cos(phi1)*(l1*sin(phi1) - l4*sin(phi4)))*((l1*sin(phi1) - l4*sin(phi4))^2 + l2^2 - l3^2 + (l1*cos(phi1) - l4*cos(phi4))^2) - 8*l1*l2^2*sin(phi1)*(l1*cos(phi1) - l4*cos(phi4)) + 8*l1*l2^2*cos(phi1)*(l1*sin(phi1) - l4*sin(phi4)))/(4*l2^2*(l1*cos(phi1) - l4*cos(phi4))^2 + 4*l2^2*(l1*sin(phi1) - l4*sin(phi4))^2 - ((l1*sin(phi1) - l4*sin(phi4))^2 + l2^2 - l3^2 + (l1*cos(phi1) - l4*cos(phi4))^2)^2)^(1/2))/2 + 2*l1*l2*sin(phi1) - 2*l1*sin(phi1)*(l1*cos(phi1) - l4*cos(phi4)) + 2*l1*cos(phi1)*(l1*sin(phi1) - l4*sin(phi4))))/(imag((4*l2^2*(l1*cos(phi1) - l4*cos(phi4))^2 + 4*l2^2*(l1*sin(phi1) - l4*sin(phi4))^2 - ((l1*sin(phi1) - l4*sin(phi4))^2 + l2^2 - l3^2 + (l1*cos(phi1) - l4*cos(phi4))^2)^2)^(1/2)) + (l1*sin(phi1) - l4*sin(phi4))^2 - 2*l2*(l1*cos(phi1) - l4*cos(phi4)) + l2^2 - l3^2 + (l1*cos(phi1) - l4*cos(phi4))^2)^2)*(imag((4*l2^2*(l1*cos(phi1) - l4*cos(phi4))^2 + 4*l2^2*(l1*sin(phi1) - l4*sin(phi4))^2 - ((l1*sin(phi1) - l4*sin(phi4))^2 + l2^2 - l3^2 + (l1*cos(phi1) - l4*cos(phi4))^2)^2)^(1/2)) + (l1*sin(phi1) - l4*sin(phi4))^2 - 2*l2*(l1*cos(phi1) - l4*cos(phi4)) + l2^2 - l3^2 + (l1*cos(phi1) - l4*cos(phi4))^2)^2)/((imag((4*l2^2*(l1*cos(phi1) - l4*cos(phi4))^2 + 4*l2^2*(l1*sin(phi1) - l4*sin(phi4))^2 - ((l1*sin(phi1) - l4*sin(phi4))^2 + l2^2 - l3^2 + (l1*cos(phi1) - l4*cos(phi4))^2)^2)^(1/2)) + (l1*sin(phi1) - l4*sin(phi4))^2 - 2*l2*(l1*cos(phi1) - l4*cos(phi4)) + l2^2 - l3^2 + (l1*cos(phi1) - l4*cos(phi4))^2)^2 + (real((4*l2^2*(l1*cos(phi1) - l4*cos(phi4))^2 + 4*l2^2*(l1*sin(phi1) - l4*sin(phi4))^2 - ((l1*sin(phi1) - l4*sin(phi4))^2 + l2^2 - l3^2 + (l1*cos(phi1) - l4*cos(phi4))^2)^2)^(1/2)) + 2*l2*(l1*sin(phi1) - l4*sin(phi4)))^2)))/(l2*cos(2*atan2(- (4*l2^2*(l1*cos(phi1) - l4*cos(phi4))^2 + 4*l2^2*(l1*sin(phi1) - l4*sin(phi4))^2 - ((l1*sin(phi1) - l4*sin(phi4))^2 + l2^2 - l3^2 + (l1*cos(phi1) - l4*cos(phi4))^2)^2)^(1/2) - 2*l2*(l1*sin(phi1) - l4*sin(phi4)), (l1*sin(phi1) - l4*sin(phi4))^2 - 2*l2*(l1*cos(phi1) - l4*cos(phi4)) + l2^2 - l3^2 + (l1*cos(phi1) - l4*cos(phi4))^2)) + l1*cos(phi1))^2))/(l4^2*((l5^2*(l2*cos(2*atan2(- (4*l2^2*(l1*cos(phi1) - l4*cos(phi4))^2 + 4*l2^2*(l1*sin(phi1) - l4*sin(phi4))^2 - ((l1*sin(phi1) - l4*sin(phi4))^2 + l2^2 - l3^2 + (l1*cos(phi1) - l4*cos(phi4))^2)^2)^(1/2) - 2*l2*(l1*sin(phi1) - l4*sin(phi4)), (l1*sin(phi1) - l4*sin(phi4))^2 - 2*l2*(l1*cos(phi1) - l4*cos(phi4)) + l2^2 - l3^2 + (l1*cos(phi1) - l4*cos(phi4))^2)) + l1*cos(phi1))^2)/l4^2 + (l5^2*(l2*sin(2*atan2(- (4*l2^2*(l1*cos(phi1) - l4*cos(phi4))^2 + 4*l2^2*(l1*sin(phi1) - l4*sin(phi4))^2 - ((l1*sin(phi1) - l4*sin(phi4))^2 + l2^2 - l3^2 + (l1*cos(phi1) - l4*cos(phi4))^2)^2)^(1/2) - 2*l2*(l1*sin(phi1) - l4*sin(phi4)), (l1*sin(phi1) - l4*sin(phi4))^2 - 2*l2*(l1*cos(phi1) - l4*cos(phi4)) + l2^2 - l3^2 + (l1*cos(phi1) - l4*cos(phi4))^2)) + l1*sin(phi1))^2)/l4^2)) + (d_phi4*l5^2*(l2*cos(2*atan2(- (4*l2^2*(l1*cos(phi1) - l4*cos(phi4))^2 + 4*l2^2*(l1*sin(phi1) - l4*sin(phi4))^2 - ((l1*sin(phi1) - l4*sin(phi4))^2 + l2^2 - l3^2 + (l1*cos(phi1) - l4*cos(phi4))^2)^2)^(1/2) - 2*l2*(l1*sin(phi1) - l4*sin(phi4)), (l1*sin(phi1) - l4*sin(phi4))^2 - 2*l2*(l1*cos(phi1) - l4*cos(phi4)) + l2^2 - l3^2 + (l1*cos(phi1) - l4*cos(phi4))^2)) + l1*cos(phi1))^2*((2*l2*cos(2*atan2(- (4*l2^2*(l1*cos(phi1) - l4*cos(phi4))^2 + 4*l2^2*(l1*sin(phi1) - l4*sin(phi4))^2 - ((l1*sin(phi1) - l4*sin(phi4))^2 + l2^2 - l3^2 + (l1*cos(phi1) - l4*cos(phi4))^2)^2)^(1/2) - 2*l2*(l1*sin(phi1) - l4*sin(phi4)), (l1*sin(phi1) - l4*sin(phi4))^2 - 2*l2*(l1*cos(phi1) - l4*cos(phi4)) + l2^2 - l3^2 + (l1*cos(phi1) - l4*cos(phi4))^2))*((real((2*(2*l4*sin(phi4)*(l1*cos(phi1) - l4*cos(phi4)) - 2*l4*cos(phi4)*(l1*sin(phi1) - l4*sin(phi4)))*((l1*sin(phi1) - l4*sin(phi4))^2 + l2^2 - l3^2 + (l1*cos(phi1) - l4*cos(phi4))^2) - 8*l2^2*l4*sin(phi4)*(l1*cos(phi1) - l4*cos(phi4)) + 8*l2^2*l4*cos(phi4)*(l1*sin(phi1) - l4*sin(phi4)))/(4*l2^2*(l1*cos(phi1) - l4*cos(phi4))^2 + 4*l2^2*(l1*sin(phi1) - l4*sin(phi4))^2 - ((l1*sin(phi1) - l4*sin(phi4))^2 + l2^2 - l3^2 + (l1*cos(phi1) - l4*cos(phi4))^2)^2)^(1/2))/2 + 2*l2*l4*cos(phi4))/(imag((4*l2^2*(l1*cos(phi1) - l4*cos(phi4))^2 + 4*l2^2*(l1*sin(phi1) - l4*sin(phi4))^2 - ((l1*sin(phi1) - l4*sin(phi4))^2 + l2^2 - l3^2 + (l1*cos(phi1) - l4*cos(phi4))^2)^2)^(1/2)) + (l1*sin(phi1) - l4*sin(phi4))^2 - 2*l2*(l1*cos(phi1) - l4*cos(phi4)) + l2^2 - l3^2 + (l1*cos(phi1) - l4*cos(phi4))^2) - ((real((4*l2^2*(l1*cos(phi1) - l4*cos(phi4))^2 + 4*l2^2*(l1*sin(phi1) - l4*sin(phi4))^2 - ((l1*sin(phi1) - l4*sin(phi4))^2 + l2^2 - l3^2 + (l1*cos(phi1) - l4*cos(phi4))^2)^2)^(1/2)) + 2*l2*(l1*sin(phi1) - l4*sin(phi4)))*(imag((2*(2*l4*sin(phi4)*(l1*cos(phi1) - l4*cos(phi4)) - 2*l4*cos(phi4)*(l1*sin(phi1) - l4*sin(phi4)))*((l1*sin(phi1) - l4*sin(phi4))^2 + l2^2 - l3^2 + (l1*cos(phi1) - l4*cos(phi4))^2) - 8*l2^2*l4*sin(phi4)*(l1*cos(phi1) - l4*cos(phi4)) + 8*l2^2*l4*cos(phi4)*(l1*sin(phi1) - l4*sin(phi4)))/(4*l2^2*(l1*cos(phi1) - l4*cos(phi4))^2 + 4*l2^2*(l1*sin(phi1) - l4*sin(phi4))^2 - ((l1*sin(phi1) - l4*sin(phi4))^2 + l2^2 - l3^2 + (l1*cos(phi1) - l4*cos(phi4))^2)^2)^(1/2))/2 + 2*l2*l4*sin(phi4) - 2*l4*sin(phi4)*(l1*cos(phi1) - l4*cos(phi4)) + 2*l4*cos(phi4)*(l1*sin(phi1) - l4*sin(phi4))))/(imag((4*l2^2*(l1*cos(phi1) - l4*cos(phi4))^2 + 4*l2^2*(l1*sin(phi1) - l4*sin(phi4))^2 - ((l1*sin(phi1) - l4*sin(phi4))^2 + l2^2 - l3^2 + (l1*cos(phi1) - l4*cos(phi4))^2)^2)^(1/2)) + (l1*sin(phi1) - l4*sin(phi4))^2 - 2*l2*(l1*cos(phi1) - l4*cos(phi4)) + l2^2 - l3^2 + (l1*cos(phi1) - l4*cos(phi4))^2)^2)*(imag((4*l2^2*(l1*cos(phi1) - l4*cos(phi4))^2 + 4*l2^2*(l1*sin(phi1) - l4*sin(phi4))^2 - ((l1*sin(phi1) - l4*sin(phi4))^2 + l2^2 - l3^2 + (l1*cos(phi1) - l4*cos(phi4))^2)^2)^(1/2)) + (l1*sin(phi1) - l4*sin(phi4))^2 - 2*l2*(l1*cos(phi1) - l4*cos(phi4)) + l2^2 - l3^2 + (l1*cos(phi1) - l4*cos(phi4))^2)^2)/((l2*cos(2*atan2(- (4*l2^2*(l1*cos(phi1) - l4*cos(phi4))^2 + 4*l2^2*(l1*sin(phi1) - l4*sin(phi4))^2 - ((l1*sin(phi1) - l4*sin(phi4))^2 + l2^2 - l3^2 + (l1*cos(phi1) - l4*cos(phi4))^2)^2)^(1/2) - 2*l2*(l1*sin(phi1) - l4*sin(phi4)), (l1*sin(phi1) - l4*sin(phi4))^2 - 2*l2*(l1*cos(phi1) - l4*cos(phi4)) + l2^2 - l3^2 + (l1*cos(phi1) - l4*cos(phi4))^2)) + l1*cos(phi1))*((imag((4*l2^2*(l1*cos(phi1) - l4*cos(phi4))^2 + 4*l2^2*(l1*sin(phi1) - l4*sin(phi4))^2 - ((l1*sin(phi1) - l4*sin(phi4))^2 + l2^2 - l3^2 + (l1*cos(phi1) - l4*cos(phi4))^2)^2)^(1/2)) + (l1*sin(phi1) - l4*sin(phi4))^2 - 2*l2*(l1*cos(phi1) - l4*cos(phi4)) + l2^2 - l3^2 + (l1*cos(phi1) - l4*cos(phi4))^2)^2 + (real((4*l2^2*(l1*cos(phi1) - l4*cos(phi4))^2 + 4*l2^2*(l1*sin(phi1) - l4*sin(phi4))^2 - ((l1*sin(phi1) - l4*sin(phi4))^2 + l2^2 - l3^2 + (l1*cos(phi1) - l4*cos(phi4))^2)^2)^(1/2)) + 2*l2*(l1*sin(phi1) - l4*sin(phi4)))^2)) + (2*l2*sin(2*atan2(- (4*l2^2*(l1*cos(phi1) - l4*cos(phi4))^2 + 4*l2^2*(l1*sin(phi1) - l4*sin(phi4))^2 - ((l1*sin(phi1) - l4*sin(phi4))^2 + l2^2 - l3^2 + (l1*cos(phi1) - l4*cos(phi4))^2)^2)^(1/2) - 2*l2*(l1*sin(phi1) - l4*sin(phi4)), (l1*sin(phi1) - l4*sin(phi4))^2 - 2*l2*(l1*cos(phi1) - l4*cos(phi4)) + l2^2 - l3^2 + (l1*cos(phi1) - l4*cos(phi4))^2))*(l2*sin(2*atan2(- (4*l2^2*(l1*cos(phi1) - l4*cos(phi4))^2 + 4*l2^2*(l1*sin(phi1) - l4*sin(phi4))^2 - ((l1*sin(phi1) - l4*sin(phi4))^2 + l2^2 - l3^2 + (l1*cos(phi1) - l4*cos(phi4))^2)^2)^(1/2) - 2*l2*(l1*sin(phi1) - l4*sin(phi4)), (l1*sin(phi1) - l4*sin(phi4))^2 - 2*l2*(l1*cos(phi1) - l4*cos(phi4)) + l2^2 - l3^2 + (l1*cos(phi1) - l4*cos(phi4))^2)) + l1*sin(phi1))*((real((2*(2*l4*sin(phi4)*(l1*cos(phi1) - l4*cos(phi4)) - 2*l4*cos(phi4)*(l1*sin(phi1) - l4*sin(phi4)))*((l1*sin(phi1) - l4*sin(phi4))^2 + l2^2 - l3^2 + (l1*cos(phi1) - l4*cos(phi4))^2) - 8*l2^2*l4*sin(phi4)*(l1*cos(phi1) - l4*cos(phi4)) + 8*l2^2*l4*cos(phi4)*(l1*sin(phi1) - l4*sin(phi4)))/(4*l2^2*(l1*cos(phi1) - l4*cos(phi4))^2 + 4*l2^2*(l1*sin(phi1) - l4*sin(phi4))^2 - ((l1*sin(phi1) - l4*sin(phi4))^2 + l2^2 - l3^2 + (l1*cos(phi1) - l4*cos(phi4))^2)^2)^(1/2))/2 + 2*l2*l4*cos(phi4))/(imag((4*l2^2*(l1*cos(phi1) - l4*cos(phi4))^2 + 4*l2^2*(l1*sin(phi1) - l4*sin(phi4))^2 - ((l1*sin(phi1) - l4*sin(phi4))^2 + l2^2 - l3^2 + (l1*cos(phi1) - l4*cos(phi4))^2)^2)^(1/2)) + (l1*sin(phi1) - l4*sin(phi4))^2 - 2*l2*(l1*cos(phi1) - l4*cos(phi4)) + l2^2 - l3^2 + (l1*cos(phi1) - l4*cos(phi4))^2) - ((real((4*l2^2*(l1*cos(phi1) - l4*cos(phi4))^2 + 4*l2^2*(l1*sin(phi1) - l4*sin(phi4))^2 - ((l1*sin(phi1) - l4*sin(phi4))^2 + l2^2 - l3^2 + (l1*cos(phi1) - l4*cos(phi4))^2)^2)^(1/2)) + 2*l2*(l1*sin(phi1) - l4*sin(phi4)))*(imag((2*(2*l4*sin(phi4)*(l1*cos(phi1) - l4*cos(phi4)) - 2*l4*cos(phi4)*(l1*sin(phi1) - l4*sin(phi4)))*((l1*sin(phi1) - l4*sin(phi4))^2 + l2^2 - l3^2 + (l1*cos(phi1) - l4*cos(phi4))^2) - 8*l2^2*l4*sin(phi4)*(l1*cos(phi1) - l4*cos(phi4)) + 8*l2^2*l4*cos(phi4)*(l1*sin(phi1) - l4*sin(phi4)))/(4*l2^2*(l1*cos(phi1) - l4*cos(phi4))^2 + 4*l2^2*(l1*sin(phi1) - l4*sin(phi4))^2 - ((l1*sin(phi1) - l4*sin(phi4))^2 + l2^2 - l3^2 + (l1*cos(phi1) - l4*cos(phi4))^2)^2)^(1/2))/2 + 2*l2*l4*sin(phi4) - 2*l4*sin(phi4)*(l1*cos(phi1) - l4*cos(phi4)) + 2*l4*cos(phi4)*(l1*sin(phi1) - l4*sin(phi4))))/(imag((4*l2^2*(l1*cos(phi1) - l4*cos(phi4))^2 + 4*l2^2*(l1*sin(phi1) - l4*sin(phi4))^2 - ((l1*sin(phi1) - l4*sin(phi4))^2 + l2^2 - l3^2 + (l1*cos(phi1) - l4*cos(phi4))^2)^2)^(1/2)) + (l1*sin(phi1) - l4*sin(phi4))^2 - 2*l2*(l1*cos(phi1) - l4*cos(phi4)) + l2^2 - l3^2 + (l1*cos(phi1) - l4*cos(phi4))^2)^2)*(imag((4*l2^2*(l1*cos(phi1) - l4*cos(phi4))^2 + 4*l2^2*(l1*sin(phi1) - l4*sin(phi4))^2 - ((l1*sin(phi1) - l4*sin(phi4))^2 + l2^2 - l3^2 + (l1*cos(phi1) - l4*cos(phi4))^2)^2)^(1/2)) + (l1*sin(phi1) - l4*sin(phi4))^2 - 2*l2*(l1*cos(phi1) - l4*cos(phi4)) + l2^2 - l3^2 + (l1*cos(phi1) - l4*cos(phi4))^2)^2)/((l2*cos(2*atan2(- (4*l2^2*(l1*cos(phi1) - l4*cos(phi4))^2 + 4*l2^2*(l1*sin(phi1) - l4*sin(phi4))^2 - ((l1*sin(phi1) - l4*sin(phi4))^2 + l2^2 - l3^2 + (l1*cos(phi1) - l4*cos(phi4))^2)^2)^(1/2) - 2*l2*(l1*sin(phi1) - l4*sin(phi4)), (l1*sin(phi1) - l4*sin(phi4))^2 - 2*l2*(l1*cos(phi1) - l4*cos(phi4)) + l2^2 - l3^2 + (l1*cos(phi1) - l4*cos(phi4))^2)) + l1*cos(phi1))^2*((imag((4*l2^2*(l1*cos(phi1) - l4*cos(phi4))^2 + 4*l2^2*(l1*sin(phi1) - l4*sin(phi4))^2 - ((l1*sin(phi1) - l4*sin(phi4))^2 + l2^2 - l3^2 + (l1*cos(phi1) - l4*cos(phi4))^2)^2)^(1/2)) + (l1*sin(phi1) - l4*sin(phi4))^2 - 2*l2*(l1*cos(phi1) - l4*cos(phi4)) + l2^2 - l3^2 + (l1*cos(phi1) - l4*cos(phi4))^2)^2 + (real((4*l2^2*(l1*cos(phi1) - l4*cos(phi4))^2 + 4*l2^2*(l1*sin(phi1) - l4*sin(phi4))^2 - ((l1*sin(phi1) - l4*sin(phi4))^2 + l2^2 - l3^2 + (l1*cos(phi1) - l4*cos(phi4))^2)^2)^(1/2)) + 2*l2*(l1*sin(phi1) - l4*sin(phi4)))^2))))/(l4^2*((l5^2*(l2*cos(2*atan2(- (4*l2^2*(l1*cos(phi1) - l4*cos(phi4))^2 + 4*l2^2*(l1*sin(phi1) - l4*sin(phi4))^2 - ((l1*sin(phi1) - l4*sin(phi4))^2 + l2^2 - l3^2 + (l1*cos(phi1) - l4*cos(phi4))^2)^2)^(1/2) - 2*l2*(l1*sin(phi1) - l4*sin(phi4)), (l1*sin(phi1) - l4*sin(phi4))^2 - 2*l2*(l1*cos(phi1) - l4*cos(phi4)) + l2^2 - l3^2 + (l1*cos(phi1) - l4*cos(phi4))^2)) + l1*cos(phi1))^2)/l4^2 + (l5^2*(l2*sin(2*atan2(- (4*l2^2*(l1*cos(phi1) - l4*cos(phi4))^2 + 4*l2^2*(l1*sin(phi1) - l4*sin(phi4))^2 - ((l1*sin(phi1) - l4*sin(phi4))^2 + l2^2 - l3^2 + (l1*cos(phi1) - l4*cos(phi4))^2)^2)^(1/2) - 2*l2*(l1*sin(phi1) - l4*sin(phi4)), (l1*sin(phi1) - l4*sin(phi4))^2 - 2*l2*(l1*cos(phi1) - l4*cos(phi4)) + l2^2 - l3^2 + (l1*cos(phi1) - l4*cos(phi4))^2)) + l1*sin(phi1))^2)/l4^2));
 
end
